simulink model "plant2016_cybership"  (R2015b)
settings: Solver=VariableStepAuto  SolverMode=SingleTasking  StartTime=0.0  StopTime=300  FixedStep=.01  RelTol=1e-3  AbsTol=1e-6
StartFcn:
  | %plot_Contr_index('open')
libraries: simulink x7
(part 2 of 2)

== system plant2016_cybership/Environment force/Wave model/2nd order Markov ==
  wn : Inport
  Gain : Gain  Gain=[omega_01^2 , 0 , 0 ; 0 , omega_02^2 , 0 ; 0 , 0 , omega_03^2]  Multiplication=Matrix(K*u) (u vector)
  Gain1 : Gain  Gain=[2*zeta_01*omega_01 , 0 , 0 ; 0 , 2*zeta_02*omega_02 , 0 ; 0 , 0 , 2*zeta_03*omega_03]  Multiplication=Matrix(K*u) (u vector)
  Integrator : Integrator  InitialCondition=[0;0;0]
  Integrator1 : Integrator  InitialCondition=[0;0;0]
  Sum1 : Sum  Inputs=-+-
  out : Outport
  wires:
  Sum1/1 -> Integrator/1
  Integrator/1 -> Integrator1/1, Gain1/1, out/1
  wn/1 -> Sum1/2
  Gain1/1 -> Sum1/3
  Integrator1/1 -> Gain/1
  Gain/1 -> Sum1/1

== system plant2016_cybership/Environment force/Environment force1/Wind direction/1st order Markov1 ==
  In1 : Inport
  2nd order LP1 : TransferFcn  Numerator=0.01^2  Denominator=[1 2*1*0.01 0.01^2]
  Constant : Constant  Value=pi*(2*rand()-1)
  Constant1 : Constant  Value=100
  Gain : Gain  Gain=2
  Sum : Sum  Inputs=|+-
  Sum1 : Sum  Inputs=++|
  Out1 : Outport
  wires:
  In1/1 -> Sum/1
  Sum/1 -> 2nd order LP1/1
  2nd order LP1/1 -> Gain/1
  Constant1/1 -> Sum1/1
  Gain/1 -> Sum1/2, Sum/2
  Sum1/1 -> Out1/1

== matlab function plant2016_cybership/Data-driven controller surge/ /MATLAB Function1 ==
  data: frs input; y output; i input; y_sqr output
function [y,y_sqr] = fcn(frs,i)
%#codegen

y       = frs(i);
y_sqr   = frs.^2;

== matlab function plant2016_cybership/Data-driven controller surge/ /MATLAB Function ==
  data: cost input; y output; i input
function y = fcn(cost,i)
%#codegen

y = cost(i);

== matlab function plant2016_cybership/Data-driven controller surge/ /Selector ==
  data: u input; y output
function y = fcn(u)
%#codegen

y = u(5);

== matlab function plant2016_cybership/Cybership II/Path calculator ==
  data: tau input; nu input; nu_dot output
function nu_dot = fcn(tau,nu)
%% Cybership I
% % % m = 14.79;
% % % Iz = 1.76;
% % % xg = 0.0375;
% % % yg = 0;
% % % 
% % % Xudot   = -2;
% % % Yvdot   = -10;
% % % Yrdot   = 0;
% % % Nrdot   = -1;
% % % 
% % % Xu      = -0.4543;
% % % Yv      = -3.083;
% % % Yr      = -7.25;
% % % Nv      = 4.1117e-4;
% % % Nr      = -1.9;
% % % 
% % % M = [m-Xudot 0 0
% % %     0 m-Yvdot m*xg-Yrdot
% % %     0 m*xg - Yrdot Iz-Nrdot];
% % % 
% % % 
% % % D = [-Xu 0 0
% % %     0 -Yv -Yr    
% % %     0 -Nv -Nr];
% % % 
% % % nu_dot = -M\D*nu + M\tau;


%% Cybership II
% Data taken from: 
% @article{RN768,
%    author = {Hassani, Vahid and Pascoal, António M. and Aguiar, A. Pedro and Athans, Michael},
%    title = {A Multiple Model Adaptive Wave Filter for Dynamic Ship Positioning},
%    journal = {IFAC Proceedings Volumes},
%    volume = {43},
%    number = {20},
%    pages = {120-125},
%    ISSN = {1474-6670},
%    DOI = {http://dx.doi.org/10.3182/20100915-3-DE-3008.00026},
%    url = {http://www.sciencedirect.com/science/article/pii/S1474667016334486},
%    year = {2010},
%    type = {Journal Article}
% }


M = [   25.8,       0,          0;
        0,          33.8,       1.0115;
        0,          1.0115,     2.76];
    
D = [   2,          0,          0;
        0,          7,          0.1;
        0,          0.1,        0.5];

nu_dot = -M\D*nu + M\tau;

end

== matlab function plant2016_cybership/Data-driven controller surge/ /MATLAB Function2 ==
  data: u input; y output
function y  = fcn(u)
y=u^2;

== matlab function plant2016_cybership/Cybership II/eta_dot ==
  data: psi input; nu input; eta_dot output
function eta_dot = fcn(psi,nu)

R = [   cos(psi)    -sin(psi)   0
        sin(psi)     cos(psi)   0
        0            0          1];

eta_dot = R*nu;

end

== matlab function plant2016_cybership/Data-driven controller sway/ /MATLAB Function ==
  data: cost input; y output; i input
function y = fcn(cost,i)
%#codegen

y = cost(i);

== matlab function plant2016_cybership/Data-driven controller sway/ /MATLAB Function1 ==
  data: frs input; y output; i input; y_sqr output
function [y,y_sqr] = fcn(frs,i)
%#codegen

y       = frs(i);
y_sqr   = frs.^2;

== matlab function plant2016_cybership/Data-driven controller sway/ /MATLAB Function2 ==
  data: u input; y output
function y  = fcn(u)
y=u^2;

== matlab function plant2016_cybership/Data-driven controller sway/ /Selector ==
  data: u input; y output
function y = fcn(u)
%#codegen

y = u(5);

== matlab function plant2016_cybership/Data-driven controller yaw/ /MATLAB Function ==
  data: cost input; y output; i input
function y = fcn(cost,i)
%#codegen

y = cost(i);

== matlab function plant2016_cybership/Data-driven controller yaw/ /MATLAB Function1 ==
  data: frs input; y output; i input; y_sqr output
function [y,y_sqr] = fcn(frs,i)
%#codegen

y       = frs(i);
y_sqr   = frs.^2;

== matlab function plant2016_cybership/Data-driven controller yaw/ /MATLAB Function2 ==
  data: u input; y output
function y  = fcn(u)
y=u^2;

== matlab function plant2016_cybership/Data-driven controller yaw/ /Selector ==
  data: u input; y output
function y = fcn(u)
%#codegen

y = u(5);

== matlab function plant2016_cybership/Environment force/Environment force1/Wind force ==
  data: beta_w input; psi input; u input; y output
function y = fcn(beta_w,psi,u)
CX = 0.80;
CY = 1.00;
CN = 0.15;

phi_w = rad2pipi(-psi+beta_w);

R = [  -CX*cos(phi_w);
        CY*sin(phi_w);
        CN*sin(2*phi_w)];

y = u.*R;

== matlab function plant2016_cybership/MATLAB Function ==
  data: eta input; y output
function y = rad2pipi(eta)

angle = eta(3);
r = rem(angle+sign(angle)*pi,2*pi);
s = sign(sign(angle) + 2*(sign(abs(rem(angle+pi,2*pi)/(2*pi)))-1));

y = [   eta(1);
        eta(2);
        r - s*pi];

== matlab function plant2016_cybership/Environment force/Environment force2/NED2Body ==
  data: psi input; u input; y output
function y = fcn(psi,u)
R = [   cos(psi)    -sin(psi)   0
        sin(psi)     cos(psi)   0
        0            0          1];

y = R\u;

== matlab function plant2016_cybership/Cybership II/MATLAB Function ==
  data: eta input; y output
function y = rad2pipi(eta)

angle = eta(3);
r = rem(angle+sign(angle)*pi,2*pi);
s = sign(sign(angle) + 2*(sign(abs(rem(angle+pi,2*pi)/(2*pi)))-1));

y = [   eta(1);
        eta(2);
        r - s*pi];
